simulink model "JenaFox_NCm_visualisation"  (R2018a)
settings: Solver=ode23s  StartTime=0.0  StopTime=20  MaxStep=maxStep  RelTol=1e-3  AbsTol=absTol
values from neighbouring files (symbols this model uses):
  amplifier = 2.28    [init_motor_parameters.m]
  c_coupling_hip = 7/hip_Ra*hip_k/hip_i    (= 1.22844788155)    [init_motor_parameters.m]
  c_coupling_knee = 7/knee_Ra*knee_k/knee_i    (= 0.698088436179)    [init_motor_parameters.m]
  c_hs = 0.1    [Fox_param.m]
  d_coupling_knee = 0.5    [init_motor_parameters.m]
  d_hs = 0.35    [Fox_param.m]
  errorswitch = true    [Fox_param.m]
  g = 9.81    [Fox_param.m]    (also in init_motor_parameters.m)
  hip_i = 1/300.4858    (= 0.00332794428223)    [init_motor_parameters.m]
  hip_Jm = 1/2*hip_m*hip_r^2    (= 1e-07)    [init_motor_parameters.m]
  hip_k = (hip_Um-hip_I0*hip_Ra)*60/(2*pi*hip_n0)    (= 0.00320895298542)    [init_motor_parameters.m]
  hip_Mrg = hip_k*hip_I0g    (= 0.000320895298542)    [init_motor_parameters.m]
  hip_Mrhg = hip_k*hip_Iag    (= 0.000381865405265)    [init_motor_parameters.m]
  hip_na = (hip_Us-(hip_I0*hip_Ra))/hip_k    (= 105.13168591)    [init_motor_parameters.m]
  hip_Ra = hip_Um/hip_Is    (= 5.49450549451)    [init_motor_parameters.m]
  IC_motor_hip_l = deg2rad(IC_phi_hip_l/hip_i)    [init_motor_parameters.m]
  IC_motor_hip_r = deg2rad(IC_phi_hip_r/hip_i)    [init_motor_parameters.m]
  IC_motor_knee_l = deg2rad(IC_phi_knee_l/knee_i)    [init_motor_parameters.m]
  IC_motor_knee_r = deg2rad(IC_phi_knee_r/knee_i)    [init_motor_parameters.m]
  IC_phi_hip_l = 10    [Fox_param.m]
  IC_phi_hip_r = -29    [Fox_param.m]
  IC_v_motor_hip = 0    [init_motor_parameters.m]
  IC_v_motor_knee = 0    [init_motor_parameters.m]
  k_gx = 10*M_RB/0.01    [Fox_param.m]
  k_gy = 150*M_RB/0.01    [Fox_param.m]
  knee_i = 1/185.8428    (= 0.00538089180748)    [init_motor_parameters.m]
  knee_Jm = 1/2*knee_m*knee_r^2    (= 3.2e-08)    [init_motor_parameters.m]
  knee_k = (knee_Um-knee_I0*knee_Ra)*60/(2*pi*knee_n0)    (= 0.000596244182085)    [init_motor_parameters.m]
  knee_Mrg = knee_k*knee_I0g    (= 6.55868600293e-05)    [init_motor_parameters.m]
  knee_Mrhg = knee_k*knee_Iag    (= 9.59953133156e-05)    [init_motor_parameters.m]
  knee_na = (knee_Us-knee_I0*knee_Ra)/knee_k    (= 1360.36733855)    [init_motor_parameters.m]
  knee_Ra = knee_Um/knee_Is    (= 1.11111111111)    [init_motor_parameters.m]
  mu_slide = 4.6    [Fox_param.m]
  mu_stick = 0.8    [Fox_param.m]
  stop5m = true    [Fox_param.m]
  v_gx_max = 0.06    [Fox_param.m]
  v_gy_max = 0.70    (= 0.7)    [Fox_param.m]
  vLimit = 0.01    [Fox_param.m]
undefined symbols (not defined in the file or in its folder): param, smiData, X, Y, Z
libraries: sm_lib x38, nesl_utility x32, simulink x22, simulink_extras x8
(part 2 of 3)

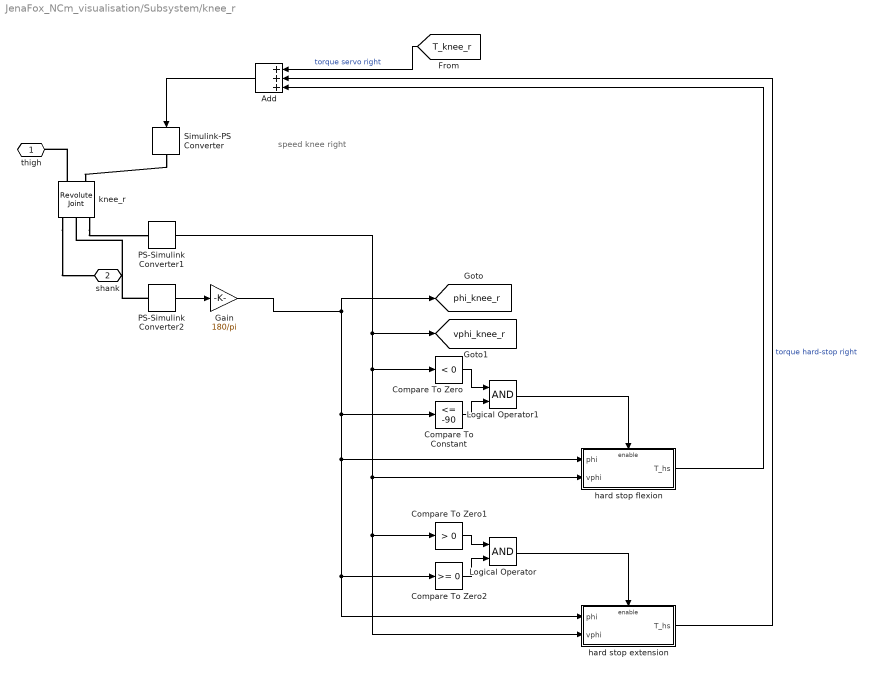
== system JenaFox_NCm_visualisation/Subsystem/knee_r ==
  note: speed knee right
  Add : Sum  Inputs=+++
  Compare To Constant : simulink/Logic and Bit Operations/Compare To Constant  relop=<=  const=-90  OutDataTypeStr=uint8
  Compare To Zero : simulink/Logic and Bit Operations/Compare To Zero  relop=<  OutDataTypeStr=uint8  ZeroCross=off
  Compare To Zero1 : simulink/Logic and Bit Operations/Compare To Zero  relop=>  OutDataTypeStr=uint8  ZeroCross=off
  Compare To Zero2 : simulink/Logic and Bit Operations/Compare To Zero  relop=>=  OutDataTypeStr=uint8
  Gain : Gain  Gain=180/pi
  Logical Operator : Logic  AllPortsSameDT=off  OutDataTypeStr=boolean
  Logical Operator1 : Logic  AllPortsSameDT=off  OutDataTypeStr=boolean
  PS-Simulink Converter1 : nesl_utility/PS-Simulink Converter  PhysicalDomain=network_engine_domain  SubClassName=ps_output  LeftPortType=input  RightPortType=output  PseudoPeriodic=off  Frequencies=[]  Unit=1  AffineConversion=off
  PS-Simulink Converter2 : nesl_utility/PS-Simulink Converter  PhysicalDomain=network_engine_domain  SubClassName=ps_output  LeftPortType=input  RightPortType=output  PseudoPeriodic=off  Frequencies=[]  Unit=1  AffineConversion=off
  Simulink-PS Converter : nesl_utility/Simulink-PS Converter  PhysicalDomain=network_engine_domain  SubClassName=ps_input  LeftPortType=input  RightPortType=output  PseudoPeriodic=off  Frequencies=[]  NoiseDistribution=none  NoiseParameters=[]  Unit=1  AffineConversion=off  FilteringAndDerivatives=provide  SimscapeFilterOrder=1  InputFilterTimeConstant=0.001  UdotUserProvided=0
  hard stop extension : Subsystem  TreatAsAtomicUnit=on
  hard stop flexion : Subsystem  TreatAsAtomicUnit=on
  knee_r : sm_lib/Joints/Revolute Joint  SenseConstraintForce=off  SenseConstraintForceX=off  SenseConstraintForceY=off  SenseConstraintForceZ=off  SenseConstraintTorque=off  SenseConstraintTorqueX=off  SenseConstraintTorqueY=off  SenseConstraintTorqueZ=off  SenseTotalForce=off  SenseTotalForceX=off  SenseTotalForceY=off  SenseTotalForceZ=off  SenseTotalTorque=off  SenseTotalTorqueX=off  SenseTotalTorqueY=off  SenseTotalTorqueZ=off  CompositeWrenchDir=FollowerOnBase  CompositeWrenchFrame=BaseFrame  EquilibriumPosition=0  EquilibriumPositionUnits=rad  SpringStiffness=0  SpringStiffnessUnits=N*m/rad  DampingCoefficient=d_joint  DampingCoefficientUnits=N*m/(rad/s)  TorqueActuationMode=InputTorque  MotionActuationMode=ComputedMotion  SensePosition=on  SenseVelocity=on  SenseAcceleration=off  SenseTorqueForce=off  PositionTargetSpecify=on  PositionTargetPriority=High  PositionTargetValue=IC_phi_knee_r  PositionTargetValueUnits=deg  VelocityTargetSpecify=off  VelocityTargetPriority=High  VelocityTargetValue=0  VelocityTargetValueUnits=deg/s
  thigh : PMIOPort  Side=Left
  shank : PMIOPort  Port=2  Side=Right
  tag scope: phi_knee_r=global, vphi_knee_r=global
  wires:
  Compare To Constant/1 -> Logical Operator1/2
  PS-Simulink Converter2/1 -> Gain/1
  hard stop extension/1(T_hs) -> Add/2  "torque hard-stop right"
  Compare To Zero1/1 -> Logical Operator/1
  Logical Operator1/1 -> hard stop flexion/Enable
  Logical Operator/1 -> hard stop extension/Enable
  Add/1 -> Simulink-PS Converter/1
  Compare To Zero/1 -> Logical Operator1/1
  PS-Simulink Converter1/1 -> [vphi_knee_r], Compare To Zero/1, hard stop flexion/2(vphi), Compare To Zero1/1, hard stop extension/2(vphi)
  hard stop flexion/1(T_hs) -> Add/3
  Compare To Zero2/1 -> Logical Operator/2
  [T_knee_r] -> Add/1  "torque servo right"
  Gain/1 -> [phi_knee_r], Compare To Constant/1, hard stop flexion/1(phi), Compare To Zero2/1, hard stop extension/1(phi)
  connections:
  Simulink-PS Converter/RConn1 -- knee_r/LConn2
  knee_r/RConn1 -- shank/RConn1
  PS-Simulink Converter2/LConn1 -- knee_r/RConn2
  knee_r/RConn3 -- PS-Simulink Converter1/LConn1
  knee_r/LConn1 -- thigh/RConn1

== system JenaFox_NCm_visualisation/Subsystem/shank_bottom_l ==
  Rigid Transform : sm_lib/Frames and Transforms/Rigid Transform  TranslationMethod=None  TranslationStandardOffset=0  TranslationLengthUnit=m  TranslationStandardAxis=+Z  TranslationCartesianOffset=[0 0 0]  TranslationROffset=0  TranslationROffsetUnits=m  TranslationZOffset=0  TranslationZOffsetUnits=m  TranslationThetaOffset=0  TranslationThetaOffsetUnits=deg  RotationMethod=AlignedAxes  RotationAngleUnits=deg  RotationStandardAxis=+Z  RotationAngle=0.0  RotationArbitraryAxis=[0 0 1]  FollAlignAxisA=+X  BaseAlignAxisA=-X  FollAlignAxisB=+Z  BaseAlignAxisB=+Y  RotationSequenceAxes=FollowerAxes  RotationSequence=XYX  RotationSequenceAngles=[0 0 0]  RotationSequenceAnglesUnits=deg  RotationMatrix=[1 0 0; 0 1 0; 0 0 1]
  Solid : sm_lib/Body Elements/Solid  InertiaType=Custom  Mass=smiData.Solid(4).mass  MassUnits=kg  CenterOfMass=smiData.Solid(4).CoM  CenterOfMassUnits=mm  MomentsOfInertia=smiData.Solid(4).MoI  MomentsOfInertiaUnits=kg*mm^2  ProductsOfInertia=smiData.Solid(4).PoI  ProductsOfInertiaUnits=kg*mm^2  DensityBased=on  Density=1000  DensityUnits=kg/m^3  DoExposeReferenceFrame=on  SerializedFrames=<Frames><Frame><Id>Frame1</Id><Value><Name>ground_contact</Name><Origin><Source>GeometricFeature</Source><FeatureName>circular curve 105</FeatureName></Origin><PrimaryAxis><DefinedDirection>+Y</DefinedDirection><Source>ReferenceFrame</Source><SourceDirection>-Y</SourceDirection><FeatureName></FeatureName></PrimaryAxis><SecondaryAxis><DefinedDirection>+X</DefinedDirection><Source>ReferenceFrame</Source><SourceDirection>+X</SourceDirection><FeatureName></FeatureName></SecondaryAxis></Value></Frame><Frame><Id>Frame2</Id><Value><Name>spring_bottom</Name><Origin><Source>GeometricFeature</Source><FeatureName>circular curve 81</FeatureName></Origin><PrimaryAxis><DefinedDirection>+Y</DefinedDirection><Source>ReferenceFrame</Source><SourceDirection>-Y</SourceDirection><FeatureName></FeatureName></PrimaryAxis><SecondaryAxis><DefinedDirection>+X</DefinedDirection><Source>ReferenceFrame</Source><SourceDirection>+X</SourceDirection><FeatureName></FeatureName></SecondaryAxis></Value></Frame></Frames>  GraphicType=FromGeometry  MarkerShape=Sphere  MarkerSize=10  GraphicVisPropType=SimpleVisualProperties  GraphicDiffuseColor=smiData.Solid(4).color  GraphicSpecularColor=[0.5 0.5 0.5 1.0]  GraphicAmbientColor=[0.15 0.15 0.15 1.0]  GraphicEmissiveColor=[0.0 0.0 0.0 1.0]  GraphicShininess=75  GraphicOpacity=smiData.Solid(4).opacity  GeometryShape=FromFile  RectangleSize=[1 1]  RectangleSizeUnits=m  BrickDimensions=[1 1 1]  BrickDimensionUnits=m  CylinderRadius=1  CylinderRadiusUnits=m  CylinderLength=1  CylinderLengthUnits=m  SphereRadius=1  SphereRadiusUnits=m  EllipsoidRadii=[1 1 1]  EllipsoidRadiiUnits=m  ExtrusionCrossSection=[1 1; -1 1; -1 -1; 1 -1]  ExtrusionCrossSectionUnits=m  ExtrusionLength=1  ExtrusionLengthUnits=m  PolygonNumSides=3  PolygonOuterRadius=1  PolygonOuterRadiusUnits=m  ExtGeomFileType=STEP  ExtGeomFileName=shank_bottom_ipt_92530788.STEP  ExtGeomFileUnits=m  RevolutionCrossSection=[1 1; 1 -1; 2 -1; 2 1]  RevolutionCrossSectionUnits=m  RevolutionExtent=Full  RevolutionAngle=180  RevolutionAngleUnits=deg
  linear elastic joint : PMIOPort  Side=Left
  toe : PMIOPort  Port=2  Side=Right
  spring_bottom : PMIOPort  Port=3  Side=Left
  connections:
  toe/RConn1 -- Solid/LConn1
  linear elastic joint/RConn1 -- Rigid Transform/RConn1 -- spring_bottom/RConn1
  Rigid Transform/LConn1 -- Solid/LConn2

== system JenaFox_NCm_visualisation/Subsystem/shank_bottom_r ==
  Rigid Transform : sm_lib/Frames and Transforms/Rigid Transform  TranslationMethod=None  TranslationStandardOffset=0  TranslationLengthUnit=m  TranslationStandardAxis=+Z  TranslationCartesianOffset=[0 0 0]  TranslationROffset=0  TranslationROffsetUnits=m  TranslationZOffset=0  TranslationZOffsetUnits=m  TranslationThetaOffset=0  TranslationThetaOffsetUnits=deg  RotationMethod=AlignedAxes  RotationAngleUnits=deg  RotationStandardAxis=+Z  RotationAngle=0.0  RotationArbitraryAxis=[0 0 1]  FollAlignAxisA=+X  BaseAlignAxisA=+X  FollAlignAxisB=+Z  BaseAlignAxisB=+Y  RotationSequenceAxes=FollowerAxes  RotationSequence=XYX  RotationSequenceAngles=[0 0 0]  RotationSequenceAnglesUnits=deg  RotationMatrix=[1 0 0; 0 1 0; 0 0 1]
  Solid : sm_lib/Body Elements/Solid  InertiaType=Custom  Mass=smiData.Solid(4).mass  MassUnits=kg  CenterOfMass=smiData.Solid(4).CoM  CenterOfMassUnits=mm  MomentsOfInertia=smiData.Solid(4).MoI  MomentsOfInertiaUnits=kg*mm^2  ProductsOfInertia=smiData.Solid(4).PoI  ProductsOfInertiaUnits=kg*mm^2  DensityBased=on  Density=1000  DensityUnits=kg/m^3  DoExposeReferenceFrame=off  SerializedFrames=<Frames><Frame><Id>Frame1</Id><Value><Name>ground_contact</Name><Origin><Source>GeometricFeature</Source><FeatureName>circular curve 105</FeatureName></Origin><PrimaryAxis><DefinedDirection>+Y</DefinedDirection><Source>ReferenceFrame</Source><SourceDirection>-Y</SourceDirection><FeatureName></FeatureName></PrimaryAxis><SecondaryAxis><DefinedDirection>+X</DefinedDirection><Source>ReferenceFrame</Source><SourceDirection>+X</SourceDirection><FeatureName></FeatureName></SecondaryAxis></Value></Frame><Frame><Id>Frame2</Id><Value><Name>spring_bottom</Name><Origin><Source>GeometricFeature</Source><FeatureName>circular curve 81</FeatureName></Origin><PrimaryAxis><DefinedDirection>+Y</DefinedDirection><Source>ReferenceFrame</Source><SourceDirection>-Y</SourceDirection><FeatureName></FeatureName></PrimaryAxis><SecondaryAxis><DefinedDirection>+X</DefinedDirection><Source>ReferenceFrame</Source><SourceDirection>+X</SourceDirection><FeatureName></FeatureName></SecondaryAxis></Value></Frame></Frames>  GraphicType=FromGeometry  MarkerShape=Sphere  MarkerSize=10  GraphicVisPropType=SimpleVisualProperties  GraphicDiffuseColor=smiData.Solid(4).color  GraphicSpecularColor=[0.5 0.5 0.5 1.0]  GraphicAmbientColor=[0.15 0.15 0.15 1.0]  GraphicEmissiveColor=[0.0 0.0 0.0 1.0]  GraphicShininess=75  GraphicOpacity=smiData.Solid(4).opacity  GeometryShape=FromFile  RectangleSize=[1 1]  RectangleSizeUnits=m  BrickDimensions=[1 1 1]  BrickDimensionUnits=m  CylinderRadius=1  CylinderRadiusUnits=m  CylinderLength=1  CylinderLengthUnits=m  SphereRadius=1  SphereRadiusUnits=m  EllipsoidRadii=[1 1 1]  EllipsoidRadiiUnits=m  ExtrusionCrossSection=[1 1; -1 1; -1 -1; 1 -1]  ExtrusionCrossSectionUnits=m  ExtrusionLength=1  ExtrusionLengthUnits=m  PolygonNumSides=3  PolygonOuterRadius=1  PolygonOuterRadiusUnits=m  ExtGeomFileType=STEP  ExtGeomFileName=shank_bottom_ipt_92530788.STEP  ExtGeomFileUnits=m  RevolutionCrossSection=[1 1; 1 -1; 2 -1; 2 1]  RevolutionCrossSectionUnits=m  RevolutionExtent=Full  RevolutionAngle=180  RevolutionAngleUnits=deg
  linear elastic joint : PMIOPort  Side=Left
  toe : PMIOPort  Port=2  Side=Right
  spring_bottom : PMIOPort  Port=3  Side=Left
  connections:
  toe/RConn1 -- Solid/LConn1
  linear elastic joint/RConn1 -- Rigid Transform/RConn1 -- spring_bottom/RConn1
  Rigid Transform/LConn1 -- Solid/RConn1

== system JenaFox_NCm_visualisation/Subsystem/shank_top_l ==
  Rigid Transform : sm_lib/Frames and Transforms/Rigid Transform  TranslationMethod=StandardAxis  TranslationStandardOffset=0.11  TranslationLengthUnit=m  TranslationStandardAxis=+Z  TranslationCartesianOffset=[0 0 0]  TranslationROffset=0  TranslationROffsetUnits=m  TranslationZOffset=0  TranslationZOffsetUnits=m  TranslationThetaOffset=0  TranslationThetaOffsetUnits=deg  RotationMethod=AlignedAxes  RotationAngleUnits=deg  RotationStandardAxis=+Z  RotationAngle=0.0  RotationArbitraryAxis=[0 0 1]  FollAlignAxisA=+X  BaseAlignAxisA=+X  FollAlignAxisB=+Y  BaseAlignAxisB=+Z  RotationSequenceAxes=FollowerAxes  RotationSequence=XYX  RotationSequenceAngles=[0 0 0]  RotationSequenceAnglesUnits=deg  RotationMatrix=[1 0 0; 0 1 0; 0 0 1]
  Solid : sm_lib/Body Elements/Solid  InertiaType=Custom  Mass=smiData.Solid(3).mass  MassUnits=kg  CenterOfMass=smiData.Solid(3).CoM  CenterOfMassUnits=mm  MomentsOfInertia=smiData.Solid(3).MoI  MomentsOfInertiaUnits=kg*mm^2  ProductsOfInertia=smiData.Solid(3).PoI  ProductsOfInertiaUnits=kg*mm^2  DensityBased=on  Density=1000  DensityUnits=kg/m^3  DoExposeReferenceFrame=off  SerializedFrames=<Frames><Frame><Id>Frame1</Id><Value><Name>spring_top</Name><Origin><Source>GeometricFeature</Source><FeatureName>circular curve 166</FeatureName></Origin><PrimaryAxis><DefinedDirection>+Y</DefinedDirection><Source>ReferenceFrame</Source><SourceDirection>-Y</SourceDirection><FeatureName></FeatureName></PrimaryAxis><SecondaryAxis><DefinedDirection>+X</DefinedDirection><Source>GeometricFeature</Source><SourceDirection>+X</SourceDirection><FeatureName>segment 110</FeatureName></SecondaryAxis></Value></Frame><Frame><Id>Frame2</Id><Value><Name>knee</Name><Origin><Source>GeometricFeature</Source><FeatureName>circular curve 135</FeatureName></Origin><PrimaryAxis><DefinedDirection>-X</DefinedDirection><Source>GeometricFeature</Source><SourceDirection>+Z</SourceDirection><FeatureName>segment 80</FeatureName></PrimaryAxis><SecondaryAxis><DefinedDirection>+Y</DefinedDirection><Source>GeometricFeature</Source><SourceDirection>+X</SourceDirection><FeatureName>segment 115</FeatureName></SecondaryAxis></Value></Frame></Frames>  GraphicType=FromGeometry  MarkerShape=Sphere  MarkerSize=10  GraphicVisPropType=SimpleVisualProperties  GraphicDiffuseColor=smiData.Solid(3).color  GraphicSpecularColor=[0.5 0.5 0.5 1.0]  GraphicAmbientColor=[0.15 0.15 0.15 1.0]  GraphicEmissiveColor=[0.0 0.0 0.0 1.0]  GraphicShininess=75  GraphicOpacity=smiData.Solid(3).opacity  GeometryShape=FromFile  RectangleSize=[1 1]  RectangleSizeUnits=m  BrickDimensions=[1 1 1]  BrickDimensionUnits=m  CylinderRadius=1  CylinderRadiusUnits=m  CylinderLength=1  CylinderLengthUnits=m  SphereRadius=1  SphereRadiusUnits=m  EllipsoidRadii=[1 1 1]  EllipsoidRadiiUnits=m  ExtrusionCrossSection=[1 1; -1 1; -1 -1; 1 -1]  ExtrusionCrossSectionUnits=m  ExtrusionLength=1  ExtrusionLengthUnits=m  PolygonNumSides=3  PolygonOuterRadius=1  PolygonOuterRadiusUnits=m  ExtGeomFileType=STEP  ExtGeomFileName=shank_top_ipt_5be12039.STEP  ExtGeomFileUnits=m  RevolutionCrossSection=[1 1; 1 -1; 2 -1; 2 1]  RevolutionCrossSectionUnits=m  RevolutionExtent=Full  RevolutionAngle=180  RevolutionAngleUnits=deg
  knee : PMIOPort  Side=Left
  linear joint : PMIOPort  Port=2  Side=Right
  spring_top : PMIOPort  Port=3  Side=Right
  connections:
  knee/RConn1 -- Solid/RConn1
  Rigid Transform/RConn1 -- spring_top/RConn1 -- Solid/LConn1
  linear joint/RConn1 -- Rigid Transform/LConn1

== system JenaFox_NCm_visualisation/Subsystem/shank_top_r ==
  Rigid Transform : sm_lib/Frames and Transforms/Rigid Transform  TranslationMethod=StandardAxis  TranslationStandardOffset=0.11  TranslationLengthUnit=m  TranslationStandardAxis=+Z  TranslationCartesianOffset=[0 0 0]  TranslationROffset=0  TranslationROffsetUnits=m  TranslationZOffset=0  TranslationZOffsetUnits=m  TranslationThetaOffset=0  TranslationThetaOffsetUnits=deg  RotationMethod=AlignedAxes  RotationAngleUnits=deg  RotationStandardAxis=+Z  RotationAngle=0.0  RotationArbitraryAxis=[0 0 1]  FollAlignAxisA=+X  BaseAlignAxisA=+X  FollAlignAxisB=+Y  BaseAlignAxisB=+Z  RotationSequenceAxes=FollowerAxes  RotationSequence=XYX  RotationSequenceAngles=[0 0 0]  RotationSequenceAnglesUnits=deg  RotationMatrix=[1 0 0; 0 1 0; 0 0 1]
  Solid : sm_lib/Body Elements/Solid  InertiaType=Custom  Mass=smiData.Solid(3).mass  MassUnits=kg  CenterOfMass=smiData.Solid(3).CoM  CenterOfMassUnits=mm  MomentsOfInertia=smiData.Solid(3).MoI  MomentsOfInertiaUnits=kg*mm^2  ProductsOfInertia=smiData.Solid(3).PoI  ProductsOfInertiaUnits=kg*mm^2  DensityBased=on  Density=1000  DensityUnits=kg/m^3  DoExposeReferenceFrame=off  SerializedFrames=<Frames><Frame><Id>Frame1</Id><Value><Name>spring_top</Name><Origin><Source>GeometricFeature</Source><FeatureName>circular curve 166</FeatureName></Origin><PrimaryAxis><DefinedDirection>+Y</DefinedDirection><Source>ReferenceFrame</Source><SourceDirection>-Y</SourceDirection><FeatureName></FeatureName></PrimaryAxis><SecondaryAxis><DefinedDirection>+X</DefinedDirection><Source>GeometricFeature</Source><SourceDirection>+X</SourceDirection><FeatureName>segment 110</FeatureName></SecondaryAxis></Value></Frame><Frame><Id>Frame2</Id><Value><Name>shank_knee_right</Name><Origin><Source>GeometricFeature</Source><FeatureName>circular curve 135</FeatureName></Origin><PrimaryAxis><DefinedDirection>+X</DefinedDirection><Source>GeometricFeature</Source><SourceDirection>+Z</SourceDirection><FeatureName>segment 110</FeatureName></PrimaryAxis><SecondaryAxis><DefinedDirection>+Y</DefinedDirection><Source>GeometricFeature</Source><SourceDirection>+X</SourceDirection><FeatureName>segment 138</FeatureName></SecondaryAxis></Value></Frame></Frames>  GraphicType=FromGeometry  MarkerShape=Sphere  MarkerSize=10  GraphicVisPropType=SimpleVisualProperties  GraphicDiffuseColor=smiData.Solid(3).color  GraphicSpecularColor=[0.5 0.5 0.5 1.0]  GraphicAmbientColor=[0.15 0.15 0.15 1.0]  GraphicEmissiveColor=[0.0 0.0 0.0 1.0]  GraphicShininess=75  GraphicOpacity=smiData.Solid(3).opacity  GeometryShape=FromFile  RectangleSize=[1 1]  RectangleSizeUnits=m  BrickDimensions=[1 1 1]  BrickDimensionUnits=m  CylinderRadius=1  CylinderRadiusUnits=m  CylinderLength=1  CylinderLengthUnits=m  SphereRadius=1  SphereRadiusUnits=m  EllipsoidRadii=[1 1 1]  EllipsoidRadiiUnits=m  ExtrusionCrossSection=[1 1; -1 1; -1 -1; 1 -1]  ExtrusionCrossSectionUnits=m  ExtrusionLength=1  ExtrusionLengthUnits=m  PolygonNumSides=3  PolygonOuterRadius=1  PolygonOuterRadiusUnits=m  ExtGeomFileType=STEP  ExtGeomFileName=shank_top_ipt_5be12039.STEP  ExtGeomFileUnits=m  RevolutionCrossSection=[1 1; 1 -1; 2 -1; 2 1]  RevolutionCrossSectionUnits=m  RevolutionExtent=Full  RevolutionAngle=180  RevolutionAngleUnits=deg
  knee : PMIOPort  Side=Left
  linear joint : PMIOPort  Port=2  Side=Right
  spring_top : PMIOPort  Port=3  Side=Right
  connections:
  knee/RConn1 -- Solid/RConn1
  Rigid Transform/RConn1 -- spring_top/RConn1 -- Solid/LConn1
  linear joint/RConn1 -- Rigid Transform/LConn1

== system JenaFox_NCm_visualisation/Subsystem/simulation terminator ==
  Clock : Clock
  PS-Simulink Converter : nesl_utility/PS-Simulink Converter  PhysicalDomain=network_engine_domain  SubClassName=ps_output  LeftPortType=input  RightPortType=output  PseudoPeriodic=off  Frequencies=[]  Unit=1  AffineConversion=off
  PS-Simulink Converter1 : nesl_utility/PS-Simulink Converter  PhysicalDomain=network_engine_domain  SubClassName=ps_output  LeftPortType=input  RightPortType=output  PseudoPeriodic=off  Frequencies=[]  Unit=1  AffineConversion=off
  PS-Simulink Converter2 : nesl_utility/PS-Simulink Converter  PhysicalDomain=network_engine_domain  SubClassName=ps_output  LeftPortType=input  RightPortType=output  PseudoPeriodic=off  Frequencies=[]  Unit=1  AffineConversion=off
  Subsystem : Subsystem
  error handling : Subsystem
  time of termination : Subsystem
  x : PMIOPort  Side=Left
  y : PMIOPort  Port=2  Side=Left
  dx : PMIOPort  Port=3  Side=Left
  wires:
  error handling/1(error) -> Subsystem/1(error), time of termination/1(error)
  PS-Simulink Converter/1 -> Subsystem/2(x), time of termination/3(x)  "x"
  PS-Simulink Converter1/1 -> error handling/3(dx)
  Clock/1 -> time of termination/2(t), error handling/1(t)
  PS-Simulink Converter2/1 -> error handling/2(y)
  connections:
  PS-Simulink Converter/LConn1 -- x/RConn1
  PS-Simulink Converter1/LConn1 -- dx/RConn1
  PS-Simulink Converter2/LConn1 -- y/RConn1

== system JenaFox_NCm_visualisation/Subsystem/thigh_l ==
  Solid : sm_lib/Body Elements/Solid  InertiaType=Custom  Mass=smiData.Solid(2).mass  MassUnits=kg  CenterOfMass=smiData.Solid(2).CoM  CenterOfMassUnits=mm  MomentsOfInertia=smiData.Solid(2).MoI  MomentsOfInertiaUnits=kg*mm^2  ProductsOfInertia=smiData.Solid(2).PoI  ProductsOfInertiaUnits=kg*mm^2  DensityBased=on  Density=1000  DensityUnits=kg/m^3  DoExposeReferenceFrame=off  SerializedFrames=<Frames><Frame><Id>Frame1</Id><Value><Name>thigh_left_knee</Name><Origin><Source>GeometricFeature</Source><FeatureName>planar surface 172</FeatureName></Origin><PrimaryAxis><DefinedDirection>+Z</DefinedDirection><Source>ReferenceFrame</Source><SourceDirection>-Y</SourceDirection><FeatureName></FeatureName></PrimaryAxis><SecondaryAxis><DefinedDirection>+X</DefinedDirection><Source>ReferenceFrame</Source><SourceDirection>+X</SourceDirection><FeatureName></FeatureName></SecondaryAxis></Value></Frame><Frame><Id>Frame2</Id><Value><Name>thigh_left_hip</Name><Origin><Source>GeometricFeature</Source><FeatureName>circular curve 156</FeatureName></Origin><PrimaryAxis><DefinedDirection>+Z</DefinedDirection><Source>ReferenceFrame</Source><SourceDirection>-Y</SourceDirection><FeatureName></FeatureName></PrimaryAxis><SecondaryAxis><DefinedDirection>+X</DefinedDirection><Source>ReferenceFrame</Source><SourceDirection>+X</SourceDirection><FeatureName></FeatureName></SecondaryAxis></Value></Frame></Frames>  GraphicType=FromGeometry  MarkerShape=Sphere  MarkerSize=10  GraphicVisPropType=SimpleVisualProperties  GraphicDiffuseColor=smiData.Solid(2).color  GraphicSpecularColor=[0.5 0.5 0.5 1.0]  GraphicAmbientColor=[0.15 0.15 0.15 1.0]  GraphicEmissiveColor=[0.0 0.0 0.0 1.0]  GraphicShininess=75  GraphicOpacity=smiData.Solid(2).opacity  GeometryShape=FromFile  RectangleSize=[1 1]  RectangleSizeUnits=m  BrickDimensions=[1 1 1]  BrickDimensionUnits=m  CylinderRadius=1  CylinderRadiusUnits=m  CylinderLength=1  CylinderLengthUnits=m  SphereRadius=1  SphereRadiusUnits=m  EllipsoidRadii=[1 1 1]  EllipsoidRadiiUnits=m  ExtrusionCrossSection=[1 1; -1 1; -1 -1; 1 -1]  ExtrusionCrossSectionUnits=m  ExtrusionLength=1  ExtrusionLengthUnits=m  PolygonNumSides=3  PolygonOuterRadius=1  PolygonOuterRadiusUnits=m  ExtGeomFileType=STEP  ExtGeomFileName=thigh_left_ipt_d01cdd9b.STEP  ExtGeomFileUnits=m  RevolutionCrossSection=[1 1; 1 -1; 2 -1; 2 1]  RevolutionCrossSectionUnits=m  RevolutionExtent=Full  RevolutionAngle=180  RevolutionAngleUnits=deg
  hip : PMIOPort  Side=Left
  knee : PMIOPort  Port=2  Side=Right
  connections:
  hip/RConn1 -- Solid/RConn1
  knee/RConn1 -- Solid/LConn1

== system JenaFox_NCm_visualisation/Subsystem/thigh_r ==
  Solid : sm_lib/Body Elements/Solid  InertiaType=Custom  Mass=smiData.Solid(2).mass  MassUnits=kg  CenterOfMass=smiData.Solid(2).CoM  CenterOfMassUnits=mm  MomentsOfInertia=smiData.Solid(2).MoI  MomentsOfInertiaUnits=kg*mm^2  ProductsOfInertia=smiData.Solid(2).PoI  ProductsOfInertiaUnits=kg*mm^2  DensityBased=on  Density=1000  DensityUnits=kg/m^3  DoExposeReferenceFrame=off  SerializedFrames=<Frames><Frame><Id>Frame1</Id><Value><Name>thigh_right_knee</Name><Origin><Source>GeometricFeature</Source><FeatureName>circular curve 616</FeatureName></Origin><PrimaryAxis><DefinedDirection>+Z</DefinedDirection><Source>ReferenceFrame</Source><SourceDirection>+Y</SourceDirection><FeatureName></FeatureName></PrimaryAxis><SecondaryAxis><DefinedDirection>+X</DefinedDirection><Source>ReferenceFrame</Source><SourceDirection>-X</SourceDirection><FeatureName></FeatureName></SecondaryAxis></Value></Frame><Frame><Id>Frame2</Id><Value><Name>thigh_right_hip</Name><Origin><Source>GeometricFeature</Source><FeatureName>circular curve 280</FeatureName></Origin><PrimaryAxis><DefinedDirection>+Z</DefinedDirection><Source>ReferenceFrame</Source><SourceDirection>+Y</SourceDirection><FeatureName></FeatureName></PrimaryAxis><SecondaryAxis><DefinedDirection>+X</DefinedDirection><Source>ReferenceFrame</Source><SourceDirection>-X</SourceDirection><FeatureName></FeatureName></SecondaryAxis></Value></Frame></Frames>  GraphicType=FromGeometry  MarkerShape=Sphere  MarkerSize=10  GraphicVisPropType=SimpleVisualProperties  GraphicDiffuseColor=smiData.Solid(2).color  GraphicSpecularColor=[0.5 0.5 0.5 1.0]  GraphicAmbientColor=[0.15 0.15 0.15 1.0]  GraphicEmissiveColor=[0.0 0.0 0.0 1.0]  GraphicShininess=75  GraphicOpacity=smiData.Solid(2).opacity  GeometryShape=FromFile  RectangleSize=[1 1]  RectangleSizeUnits=m  BrickDimensions=[1 1 1]  BrickDimensionUnits=m  CylinderRadius=1  CylinderRadiusUnits=m  CylinderLength=1  CylinderLengthUnits=m  SphereRadius=1  SphereRadiusUnits=m  EllipsoidRadii=[1 1 1]  EllipsoidRadiiUnits=m  ExtrusionCrossSection=[1 1; -1 1; -1 -1; 1 -1]  ExtrusionCrossSectionUnits=m  ExtrusionLength=1  ExtrusionLengthUnits=m  PolygonNumSides=3  PolygonOuterRadius=1  PolygonOuterRadiusUnits=m  ExtGeomFileType=STEP  ExtGeomFileName=thigh_left_ipt_d01cdd9b.STEP  ExtGeomFileUnits=m  RevolutionCrossSection=[1 1; 1 -1; 2 -1; 2 1]  RevolutionCrossSectionUnits=m  RevolutionExtent=Full  RevolutionAngle=180  RevolutionAngleUnits=deg
  hip : PMIOPort  Side=Left
  knee : PMIOPort  Port=2  Side=Right
  connections:
  knee/RConn1 -- Solid/LConn1
  Solid/RConn1 -- hip/RConn1

== system JenaFox_NCm_visualisation/Subsystem/trunk ==
  Solid : sm_lib/Body Elements/Solid  InertiaType=Custom  Mass=smiData.Solid(1).mass  MassUnits=kg  CenterOfMass=smiData.Solid(1).CoM  CenterOfMassUnits=mm  MomentsOfInertia=smiData.Solid(1).MoI  MomentsOfInertiaUnits=kg*mm^2  ProductsOfInertia=smiData.Solid(1).PoI  ProductsOfInertiaUnits=kg*mm^2  DensityBased=on  Density=1000  DensityUnits=kg/m^3  DoExposeReferenceFrame=off  SerializedFrames=<Frames><Frame><Id>Frame1</Id><Value><Name>hip_right</Name><Origin><Source>GeometricFeature</Source><FeatureName>circular curve 591</FeatureName></Origin><PrimaryAxis><DefinedDirection>+Z</DefinedDirection><Source>ReferenceFrame</Source><SourceDirection>+X</SourceDirection><FeatureName></FeatureName></PrimaryAxis><SecondaryAxis><DefinedDirection>+X</DefinedDirection><Source>ReferenceFrame</Source><SourceDirection>-Z</SourceDirection><FeatureName></FeatureName></SecondaryAxis></Value></Frame><Frame><Id>Frame2</Id><Value><Name>hip_left</Name><Origin><Source>GeometricFeature</Source><FeatureName>circular curve 612</FeatureName></Origin><PrimaryAxis><DefinedDirection>+Z</DefinedDirection><Source>ReferenceFrame</Source><SourceDirection>+X</SourceDirection><FeatureName></FeatureName></PrimaryAxis><SecondaryAxis><DefinedDirection>+X</DefinedDirection><Source>ReferenceFrame</Source><SourceDirection>-Z</SourceDirection><FeatureName></FeatureName></SecondaryAxis></Value></Frame><Frame><Id>Frame3</Id><Value><Name>boom_connector</Name><Origin><Source>GeometricFeature</Source><FeatureName>circular curve 1475</FeatureName></Origin><PrimaryAxis><DefinedDirection>+X</DefinedDirection><Source>ReferenceFrame</Source><SourceDirection>-Z</SourceDirection><FeatureName></FeatureName></PrimaryAxis><SecondaryAxis><DefinedDirection>+Y</DefinedDirection><Source>ReferenceFrame</Source><SourceDirection>+Y</SourceDirection><FeatureName></FeatureName></SecondaryAxis></Value></Frame></Frames>  GraphicType=FromGeometry  MarkerShape=Sphere  MarkerSize=10  GraphicVisPropType=SimpleVisualProperties  GraphicDiffuseColor=smiData.Solid(1).color  GraphicSpecularColor=[0.5 0.5 0.5 1.0]  GraphicAmbientColor=[0.15 0.15 0.15 1.0]  GraphicEmissiveColor=[0.0 0.0 0.0 1.0]  GraphicShininess=75  GraphicOpacity=smiData.Solid(1).opacity  GeometryShape=FromFile  RectangleSize=[1 1]  RectangleSizeUnits=m  BrickDimensions=[1 1 1]  BrickDimensionUnits=m  CylinderRadius=1  CylinderRadiusUnits=m  CylinderLength=1  CylinderLengthUnits=m  SphereRadius=1  SphereRadiusUnits=m  EllipsoidRadii=[1 1 1]  EllipsoidRadiiUnits=m  ExtrusionCrossSection=[1 1; -1 1; -1 -1; 1 -1]  ExtrusionCrossSectionUnits=m  ExtrusionLength=1  ExtrusionLengthUnits=m  PolygonNumSides=3  PolygonOuterRadius=1  PolygonOuterRadiusUnits=m  ExtGeomFileType=STEP  ExtGeomFileName=trunk_ipt_7785b5f2.STEP  ExtGeomFileUnits=m  RevolutionCrossSection=[1 1; 1 -1; 2 -1; 2 1]  RevolutionCrossSectionUnits=m  RevolutionExtent=Full  RevolutionAngle=180  RevolutionAngleUnits=deg
  hip left : PMIOPort  Side=Right
  hip right : PMIOPort  Port=2  Side=Right
  boom : PMIOPort  Port=3  Side=Left
  connections:
  Solid/RConn1 -- hip left/RConn1
  hip right/RConn1 -- Solid/LConn1
  boom/RConn1 -- Solid/LConn2

== system JenaFox_NCm_visualisation/motor model/hip_motor_left ==
  note: IC_phi_motor
  note: IC_v_motor
  note: due to neglectible inductivity the
      | PT1 - transfer function is reduced to an
      | proportional transfer function
      | (Modellbildung und Simulation dynamischer Systeme, S.122)
  U : Inport
  phi_motor : Inport  Port=2
  Add1 : Sum  Inputs=+--
  M_func_hip1 : Lookup  InputValues=[-10^10 -hip_na -0.001 0 0.001 hip_na 10^10]  Table=[-hip_Mrg -hip_Mrg -hip_Mrhg 0 hip_Mrhg hip_Mrg hip_Mrg]
  Radians to Degrees : simulink_extras/Transformations/Radians to Degrees
  Sum1 : Sum  Inputs=|+-
  elastic coupling : Sum  Inputs=+-
  elasticity : Gain  Gain=c_coupling_hip
  gearhead : Gain  Gain=hip_i
  gearhead1 : Gain  Gain=hip_i
  motor constant 1 : Gain  Gain=hip_k
  motor constant1 : Gain  Gain=hip_k
  motor interia : Gain  Gain=1/hip_Jm
  position : Integrator  InitialCondition=IC_motor_hip_l  ContinuousStateAttributes='position_hip'
  rotor resistor1 : Gain  Gain=1/hip_Ra
  speed : Integrator  InitialCondition=IC_v_motor_hip  ContinuousStateAttributes='speed_hip'
  motor_torque : Outport
  current : Outport  Port=2
  wires:
  elasticity/1 -> motor_torque/1, gearhead1/1  "coupling torque"
  gearhead1/1 -> Add1/3
  phi_motor/1 -> elastic coupling/2
  U/1 -> Sum1/1
  Radians to Degrees/1 -> gearhead/1  "position in °"
  gearhead/1 -> elastic coupling/1
  elastic coupling/1 -> elasticity/1
  position/1 -> Radians to Degrees/1  "position"
  motor constant 1/1 -> Sum1/2  "inductive voltage"
  speed/1 -> motor constant 1/1, M_func_hip1/1, position/1  "motor speed"
  Sum1/1 -> rotor resistor1/1
  motor interia/1 -> speed/1  "acceleration"
  Add1/1 -> motor interia/1
  M_func_hip1/1 -> Add1/2  "friction torque"
  motor constant1/1 -> Add1/1  "motor torque"
  rotor resistor1/1 -> current/1, motor constant1/1  "current"

== system JenaFox_NCm_visualisation/motor model/hip_motor_right ==
  note: IC_phi_motor
  note: IC_v_motor
  note: due to neglectible inductivity the
      | PT1 - transfer function is reduced to an
      | proportional transfer function
      | (Modellbildung und Simulation dynamischer Systeme, S.122)
  U : Inport
  phi_motor : Inport  Port=2
  Add1 : Sum  Inputs=+--
  M_func_hip1 : Lookup  InputValues=[-10^10 -hip_na -0.001 0 0.001 hip_na 10^10]  Table=[-hip_Mrg -hip_Mrg -hip_Mrhg 0 hip_Mrhg hip_Mrg hip_Mrg]
  Radians to Degrees : simulink_extras/Transformations/Radians to Degrees
  Sum1 : Sum  Inputs=|+-
  elastic coupling : Sum  Inputs=+-
  elasticity : Gain  Gain=c_coupling_hip
  gearhead : Gain  Gain=hip_i
  gearhead1 : Gain  Gain=hip_i
  motor constant 1 : Gain  Gain=hip_k
  motor constant1 : Gain  Gain=hip_k
  motor interia : Gain  Gain=1/hip_Jm
  position : Integrator  InitialCondition=IC_motor_hip_r  ContinuousStateAttributes='position_hip'
  rotor resistor1 : Gain  Gain=1/hip_Ra
  speed : Integrator  InitialCondition=IC_v_motor_hip  ContinuousStateAttributes='speed_hip'
  motor_torque : Outport
  current : Outport  Port=2
  wires:
  elasticity/1 -> motor_torque/1, gearhead1/1  "coupling torque"
  gearhead1/1 -> Add1/3
  phi_motor/1 -> elastic coupling/2
  U/1 -> Sum1/1
  Radians to Degrees/1 -> gearhead/1  "position in °"
  gearhead/1 -> elastic coupling/1
  elastic coupling/1 -> elasticity/1
  position/1 -> Radians to Degrees/1  "position"
  motor constant 1/1 -> Sum1/2  "inductive voltage"
  speed/1 -> motor constant 1/1, M_func_hip1/1, position/1  "motor speed"
  Sum1/1 -> rotor resistor1/1
  motor interia/1 -> speed/1  "acceleration"
  Add1/1 -> motor interia/1
  M_func_hip1/1 -> Add1/2  "friction torque"
  motor constant1/1 -> Add1/1  "motor torque"
  rotor resistor1/1 -> current/1, motor constant1/1  "current"

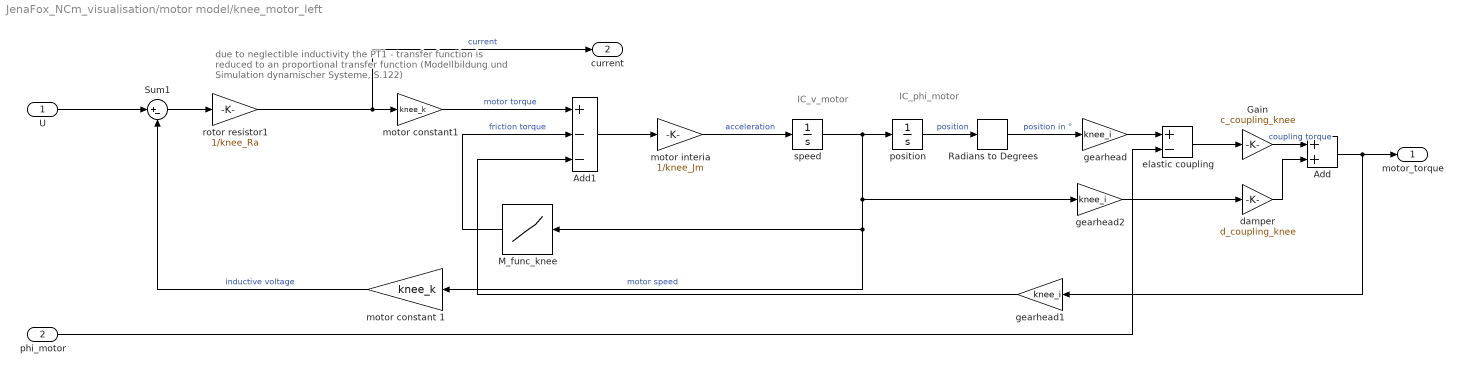
== system JenaFox_NCm_visualisation/motor model/knee_motor_left ==
  note: due to neglectible inductivity the
      | PT1 - transfer function is reduced to an
      | proportional transfer function
      | (Modellbildung und Simulation dynamischer Systeme, S.122)
  note: IC_v_motor
  note: IC_phi_motor
  U : Inport
  phi_motor : Inport  Port=2
  Add : Sum
  Add1 : Sum  Inputs=+--
  Gain : Gain  Gain=c_coupling_knee
  M_func_knee : Lookup  InputValues=[-10^10 -knee_na -0.001 0 0.001 knee_na 10^10]  Table=[-knee_Mrg -knee_Mrg -knee_Mrhg 0 knee_Mrhg knee_Mrg knee_Mrg]
  Radians to Degrees : simulink_extras/Transformations/Radians to Degrees
  Sum1 : Sum  Inputs=|+-
  damper : Gain  Gain=d_coupling_knee
  elastic coupling : Sum  Inputs=+-
  gearhead : Gain  Gain=knee_i
  gearhead1 : Gain  Gain=knee_i
  gearhead2 : Gain  Gain=knee_i
  motor constant 1 : Gain  Gain=knee_k
  motor constant1 : Gain  Gain=knee_k
  motor interia : Gain  Gain=1/knee_Jm
  position : Integrator  InitialCondition=IC_motor_knee_l  ContinuousStateAttributes='position_hip'
  rotor resistor1 : Gain  Gain=1/knee_Ra
  speed : Integrator  InitialCondition=IC_v_motor_knee  ContinuousStateAttributes='speed_hip'
  motor_torque : Outport
  current : Outport  Port=2
  wires:
  gearhead1/1 -> Add1/3
  rotor resistor1/1 -> motor constant1/1, current/1  "current"
  motor constant1/1 -> Add1/1  "motor torque"
  M_func_knee/1 -> Add1/2  "friction torque"
  Add1/1 -> motor interia/1
  motor interia/1 -> speed/1  "acceleration"
  Sum1/1 -> rotor resistor1/1
  speed/1 -> position/1, M_func_knee/1, motor constant 1/1, gearhead2/1  "motor speed"
  position/1 -> Radians to Degrees/1  "position"
  elastic coupling/1 -> Gain/1
  gearhead/1 -> elastic coupling/1
  Radians to Degrees/1 -> gearhead/1  "position in °"
  U/1 -> Sum1/1
  phi_motor/1 -> elastic coupling/2
  motor constant 1/1 -> Sum1/2  "inductive voltage"
  Gain/1 -> Add/1  "coupling torque"
  Add/1 -> motor_torque/1, gearhead1/1
  gearhead2/1 -> damper/1
  damper/1 -> Add/2

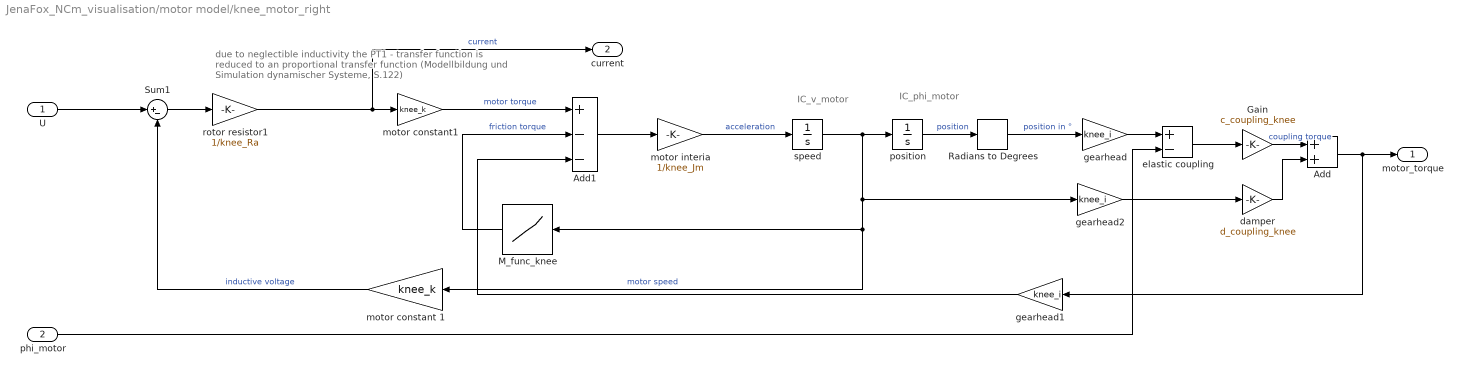
== system JenaFox_NCm_visualisation/motor model/knee_motor_right ==
  note: due to neglectible inductivity the
      | PT1 - transfer function is reduced to an
      | proportional transfer function
      | (Modellbildung und Simulation dynamischer Systeme, S.122)
  note: IC_v_motor
  note: IC_phi_motor
  U : Inport
  phi_motor : Inport  Port=2
  Add : Sum
  Add1 : Sum  Inputs=+--
  Gain : Gain  Gain=c_coupling_knee
  M_func_knee : Lookup  InputValues=[-10^10 -knee_na -0.001 0 0.001 knee_na 10^10]  Table=[-knee_Mrg -knee_Mrg -knee_Mrhg 0 knee_Mrhg knee_Mrg knee_Mrg]
  Radians to Degrees : simulink_extras/Transformations/Radians to Degrees
  Sum1 : Sum  Inputs=|+-
  damper : Gain  Gain=d_coupling_knee
  elastic coupling : Sum  Inputs=+-
  gearhead : Gain  Gain=knee_i
  gearhead1 : Gain  Gain=knee_i
  gearhead2 : Gain  Gain=knee_i
  motor constant 1 : Gain  Gain=knee_k
  motor constant1 : Gain  Gain=knee_k
  motor interia : Gain  Gain=1/knee_Jm
  position : Integrator  InitialCondition=IC_phi_motor_knee  ContinuousStateAttributes='position_hip'
  rotor resistor1 : Gain  Gain=1/knee_Ra
  speed : Integrator  InitialCondition=IC_v_motor_knee  ContinuousStateAttributes='speed_hip'
  motor_torque : Outport
  current : Outport  Port=2
  wires:
  gearhead1/1 -> Add1/3
  rotor resistor1/1 -> motor constant1/1, current/1  "current"
  motor constant1/1 -> Add1/1  "motor torque"
  M_func_knee/1 -> Add1/2  "friction torque"
  Add1/1 -> motor interia/1
  motor interia/1 -> speed/1  "acceleration"
  Sum1/1 -> rotor resistor1/1
  speed/1 -> position/1, M_func_knee/1, motor constant 1/1, gearhead2/1  "motor speed"
  position/1 -> Radians to Degrees/1  "position"
  elastic coupling/1 -> Gain/1
  gearhead/1 -> elastic coupling/1
  Radians to Degrees/1 -> gearhead/1  "position in °"
  U/1 -> Sum1/1
  phi_motor/1 -> elastic coupling/2
  motor constant 1/1 -> Sum1/2  "inductive voltage"
  Gain/1 -> Add/1  "coupling torque"
  Add/1 -> motor_torque/1, gearhead1/1
  gearhead2/1 -> damper/1
  damper/1 -> Add/2

== system JenaFox_NCm_visualisation/Subsystem/Ground Contact Model/Ground Friction Model ==
  note: Horizontal Ground Friction Model
  note: Vertical Ground Stiction Model
  dy [m] : Inport
  vy [m/s] : Inport  Port=2
  x [m] : Inport  Port=3
  vx [m/s] : Inport  Port=4
  Contact! : EnablePort  StatesWhenEnabling=reset  PropagateVarSize=During execution
  Data Type Conversion : DataTypeConversion  OutDataTypeStr=double
  Friction Switch : Subsystem
  Gain3 : Gain  Gain=k_gy
  Gain4 : Gain  Gain=1/v_gy_max
  Logical Operator : Logic  Operator=NOT  AllPortsSameDT=off  OutDataTypeStr=boolean
  Mux1 : Mux  Inputs=2
  Sum1 : Sum
  X-Axis Kinetic Friction Model : Subsystem
  X-Axis Static Friction Model : Subsystem
  Y-Axis Ground Force : Fcn  Expr="- u(1)  *  (1-u(2)) * (u(2)<1)"
  Fy_Ground[N] : Outport  OutputWhenDisabled=reset  InitialOutput=0
      settings: AttributesFormatString=initial = '%<InitialOutput>'\nwhen disabled = '%<OutputWhenDisabled>'
  Fx_Friction [N] : Outport  Port=2  OutputWhenDisabled=reset  InitialOutput=0
      settings: AttributesFormatString=initial = '%<InitialOutput>'\nwhen\ndisabled\n'%<OutputWhenDisabled>'
  Stiction! : Outport  Port=3  OutputWhenDisabled=reset  InitialOutput=0
      settings: AttributesFormatString=initial = '%<InitialOutput>'\nwhen\ndisabled\n'%<OutputWhenDisabled>'
  wires:
  dy [m]/1 -> Gain3/1
  vy [m/s]/1 -> Gain4/1
  x [m]/1 -> X-Axis Static Friction Model/2(pos [m]), X-Axis Kinetic Friction Model/1(pos [m])
  vx [m/s]/1 -> X-Axis Static Friction Model/3(vel [m/s]), X-Axis Kinetic Friction Model/2(vel [m/s])
  X-Axis Kinetic Friction Model/1(posFP [m]) -> X-Axis Static Friction Model/4(posFP [m])
  X-Axis Kinetic Friction Model/3(F_Slide [N]) -> Sum1/2
  X-Axis Static Friction Model/1(F_Stick [N]) -> Sum1/1
  Sum1/1 -> Fx_Friction [N]/1
  Friction Switch/1(Stiction) -> X-Axis Static Friction Model/Enable, Logical Operator/1, Data Type Conversion/1
  X-Axis Static Friction Model/2(Sliding!) -> Friction Switch/1(Slide!)
  X-Axis Kinetic Friction Model/2(Stiction!) -> Friction Switch/2(Stick!)
  Logical Operator/1 -> X-Axis Kinetic Friction Model/Enable
  Data Type Conversion/1 -> Stiction!/1
  Mux1/1 -> Y-Axis Ground Force/1
  Gain3/1 -> Mux1/1
  Gain4/1 -> Mux1/2
  Y-Axis Ground Force/1 -> Fy_Ground[N]/1, X-Axis Static Friction Model/1(F_Normal [N]), X-Axis Kinetic Friction Model/3(F_Normal [N])

== system JenaFox_NCm_visualisation/Subsystem/Ground Contact Model1/Ground Friction Model ==
  note: Horizontal Ground Friction Model
  note: Vertical Ground Stiction Model
  dy [m] : Inport
  vy [m/s] : Inport  Port=2
  x [m] : Inport  Port=3
  vx [m/s] : Inport  Port=4
  Contact! : EnablePort  StatesWhenEnabling=reset  PropagateVarSize=During execution
  Data Type Conversion : DataTypeConversion  OutDataTypeStr=double
  Friction Switch : Subsystem
  Gain3 : Gain  Gain=k_gy
  Gain4 : Gain  Gain=1/v_gy_max
  Logical Operator : Logic  Operator=NOT  AllPortsSameDT=off  OutDataTypeStr=boolean
  Mux1 : Mux  Inputs=2
  Sum1 : Sum
  X-Axis Kinetic Friction Model : Subsystem
  X-Axis Static Friction Model : Subsystem
  Y-Axis Ground Force : Fcn  Expr="- u(1)  *  (1-u(2)) * (u(2)<1)"
  Fy_Ground[N] : Outport  OutputWhenDisabled=reset  InitialOutput=0
      settings: AttributesFormatString=initial = '%<InitialOutput>'\nwhen disabled = '%<OutputWhenDisabled>'
  Fx_Friction [N] : Outport  Port=2  OutputWhenDisabled=reset  InitialOutput=0
      settings: AttributesFormatString=initial = '%<InitialOutput>'\nwhen\ndisabled\n'%<OutputWhenDisabled>'
  Stiction! : Outport  Port=3  OutputWhenDisabled=reset  InitialOutput=0
      settings: AttributesFormatString=initial = '%<InitialOutput>'\nwhen\ndisabled\n'%<OutputWhenDisabled>'
  wires:
  dy [m]/1 -> Gain3/1
  vy [m/s]/1 -> Gain4/1
  x [m]/1 -> X-Axis Static Friction Model/2(pos [m]), X-Axis Kinetic Friction Model/1(pos [m])
  vx [m/s]/1 -> X-Axis Static Friction Model/3(vel [m/s]), X-Axis Kinetic Friction Model/2(vel [m/s])
  X-Axis Kinetic Friction Model/1(posFP [m]) -> X-Axis Static Friction Model/4(posFP [m])
  X-Axis Kinetic Friction Model/3(F_Slide [N]) -> Sum1/2
  X-Axis Static Friction Model/1(F_Stick [N]) -> Sum1/1
  Sum1/1 -> Fx_Friction [N]/1
  Friction Switch/1(Stiction) -> X-Axis Static Friction Model/Enable, Logical Operator/1, Data Type Conversion/1
  X-Axis Static Friction Model/2(Sliding!) -> Friction Switch/1(Slide!)
  X-Axis Kinetic Friction Model/2(Stiction!) -> Friction Switch/2(Stick!)
  Logical Operator/1 -> X-Axis Kinetic Friction Model/Enable
  Data Type Conversion/1 -> Stiction!/1
  Mux1/1 -> Y-Axis Ground Force/1
  Gain3/1 -> Mux1/1
  Gain4/1 -> Mux1/2
  Y-Axis Ground Force/1 -> Fy_Ground[N]/1, X-Axis Static Friction Model/1(F_Normal [N]), X-Axis Kinetic Friction Model/3(F_Normal [N])

== system JenaFox_NCm_visualisation/Subsystem/knee_l/hard stop extension ==
  note: generate a positive torque to counteract flexion
      | beyond -90°
      | and negative torque to inhibit hyperextension beyond 0°
  phi : Inport
  vphi : Inport  Port=2
  Enable : EnablePort  PropagateVarSize=During execution
  Fcn : Fcn  Expr=c_hs*(0-u[1])-d_hs*u[2]
  Mux : Mux  Inputs=2
  T_hs : Outport  OutputWhenDisabled=reset  InitialOutput=0
  wires:
  phi/1 -> Mux/1
  vphi/1 -> Mux/2
  Mux/1 -> Fcn/1
  Fcn/1 -> T_hs/1

== system JenaFox_NCm_visualisation/Subsystem/knee_l/hard stop flexion ==
  note: generate a positive torque to counteract flexion
      | beyond -90°
      | and negative torque to inhibit hyperextension beyond 0°
  phi : Inport
  vphi : Inport  Port=2
  Enable : EnablePort  PropagateVarSize=During execution
  Fcn : Fcn  Expr=c_hs*(-92-u[1])-d_hs*u[2]
  Mux : Mux  Inputs=2
  T_hs : Outport  OutputWhenDisabled=reset  InitialOutput=0
  wires:
  Fcn/1 -> T_hs/1
  Mux/1 -> Fcn/1
  vphi/1 -> Mux/2
  phi/1 -> Mux/1

== system JenaFox_NCm_visualisation/Subsystem/knee_r/hard stop extension ==
  note: generate a positive torque to counteract flexion
      | beyond -90°
      | and negative torque to inhibit hyperextension beyond 0°
  phi : Inport
  vphi : Inport  Port=2
  Enable : EnablePort  PropagateVarSize=During execution
  Fcn : Fcn  Expr=c_hs*(0-u[1])-d_hs*u[2]
  Mux : Mux  Inputs=2
  T_hs : Outport  OutputWhenDisabled=reset  InitialOutput=0
  wires:
  phi/1 -> Mux/1
  vphi/1 -> Mux/2
  Mux/1 -> Fcn/1
  Fcn/1 -> T_hs/1

== system JenaFox_NCm_visualisation/Subsystem/knee_r/hard stop flexion ==
  note: generate a positive torque to counteract flexion
      | beyond -90°
      | and negative torque to inhibit hyperextension beyond 0°
  phi : Inport
  vphi : Inport  Port=2
  Enable : EnablePort  PropagateVarSize=During execution
  Fcn : Fcn  Expr=c_hs*(-92-u[1])-d_hs*u[2]
  Mux : Mux  Inputs=2
  T_hs : Outport  OutputWhenDisabled=reset  InitialOutput=0
  wires:
  Fcn/1 -> T_hs/1
  Mux/1 -> Fcn/1
  vphi/1 -> Mux/2
  phi/1 -> Mux/1

== system JenaFox_NCm_visualisation/Subsystem/simulation terminator/Subsystem ==
  error : Inport
  x : Inport  Port=2
  Compare To Constant5 : simulink/Logic and Bit Operations/Compare To Constant  relop=>=  const=5  OutDataTypeStr=boolean
  Constant : Constant  Value=errorswitch
  Constant1 : Constant  Value=stop5m
  Logical Operator : Logic  Operator=OR  AllPortsSameDT=off  OutDataTypeStr=boolean
  Logical Operator1 : Logic  AllPortsSameDT=off  OutDataTypeStr=boolean
  Logical Operator2 : Logic  AllPortsSameDT=off  OutDataTypeStr=boolean
  Stop Simulation1 : Stop
  wires:
  x/1 -> Compare To Constant5/1
  Logical Operator2/1 -> Logical Operator/2
  Constant/1 -> Logical Operator1/1
  error/1 -> Logical Operator1/2
  Logical Operator1/1 -> Logical Operator/1
  Logical Operator/1 -> Stop Simulation1/1
  Constant1/1 -> Logical Operator2/1
  Compare To Constant5/1 -> Logical Operator2/2

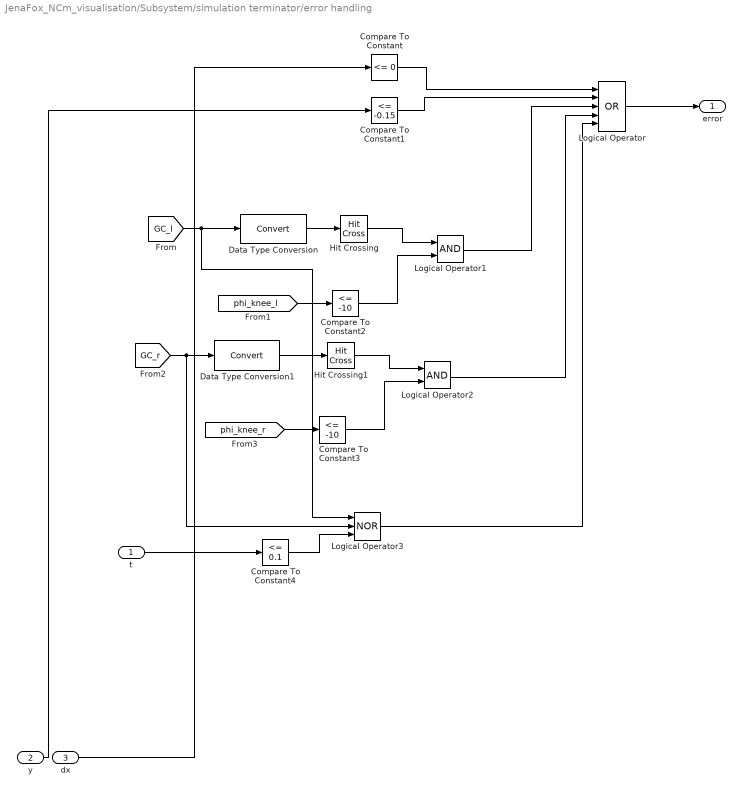
== system JenaFox_NCm_visualisation/Subsystem/simulation terminator/error handling ==
  t : Inport
  y : Inport  Port=2
  dx : Inport  Port=3
  Compare To Constant : simulink/Logic and Bit Operations/Compare To Constant  relop=<=  const=0  OutDataTypeStr=boolean
  Compare To Constant1 : simulink/Logic and Bit Operations/Compare To Constant  relop=<=  const=-0.15  OutDataTypeStr=boolean
  Compare To Constant2 : simulink/Logic and Bit Operations/Compare To Constant  relop=<=  const=-10  OutDataTypeStr=boolean
  Compare To Constant3 : simulink/Logic and Bit Operations/Compare To Constant  relop=<=  const=-10  OutDataTypeStr=boolean
  Compare To Constant4 : simulink/Logic and Bit Operations/Compare To Constant  relop=<=  const=0.1  OutDataTypeStr=boolean
  Data Type Conversion : DataTypeConversion
  Data Type Conversion1 : DataTypeConversion
  Hit Crossing : HitCross  HitCrossingOffset=0.5  HitCrossingDirection=rising
  Hit Crossing1 : HitCross  HitCrossingOffset=0.5  HitCrossingDirection=rising
  Logical Operator : Logic  Operator=OR  Inputs=5  AllPortsSameDT=off  OutDataTypeStr=boolean
  Logical Operator1 : Logic  AllPortsSameDT=off  OutDataTypeStr=boolean
  Logical Operator2 : Logic  AllPortsSameDT=off  OutDataTypeStr=boolean
  Logical Operator3 : Logic  Operator=NOR  Inputs=3  AllPortsSameDT=off  OutDataTypeStr=boolean
  error : Outport
  wires:
  [phi_knee_r] -> Compare To Constant3/1
  [GC_r] -> Logical Operator3/2, Data Type Conversion1/1
  Compare To Constant3/1 -> Logical Operator2/2
  Logical Operator1/1 -> Logical Operator/3
  Hit Crossing/1 -> Logical Operator1/1
  Logical Operator3/1 -> Logical Operator/5
  Compare To Constant2/1 -> Logical Operator1/2
  [phi_knee_l] -> Compare To Constant2/1
  Hit Crossing1/1 -> Logical Operator2/1
  Data Type Conversion1/1 -> Hit Crossing1/1
  y/1 -> Compare To Constant1/1
  t/1 -> Compare To Constant4/1
  Logical Operator2/1 -> Logical Operator/4
  Data Type Conversion/1 -> Hit Crossing/1
  Compare To Constant4/1 -> Logical Operator3/3
  [GC_l] -> Logical Operator3/1, Data Type Conversion/1
  Logical Operator/1 -> error/1
  Compare To Constant1/1 -> Logical Operator/2
  dx/1 -> Compare To Constant/1
  Compare To Constant/1 -> Logical Operator/1

== system JenaFox_NCm_visualisation/Subsystem/simulation terminator/time of termination ==
  error : Inport
  t : Inport  Port=2
  x : Inport  Port=3
  Divide : Product  Inputs=*/
  Gain : Gain  Gain=5
  Mux1 : Mux  Inputs=2
  Switch : Switch  Criteria=u2 > Threshold  Threshold=0.5
  To Workspace : ToWorkspace  VariableName=t_end  SampleTime=-1
      settings: MaxDataPoints=1
  wires:
  x/1 -> Divide/2, Mux1/2
  error/1 -> Switch/2
  t/1 -> Switch/3, Gain/1
  Mux1/1 -> To Workspace/1
  Gain/1 -> Divide/1
  Switch/1 -> Mux1/1
  Divide/1 -> Switch/1

== system JenaFox_NCm_visualisation/Subsystem/Ground Contact Model/Ground Friction Model/Friction Switch ==
  note: Static/Kinetic Friction Switch
  Slide! : Inport
  Stick! : Inport  Port=2
  Memory : Memory
  S-R Flip-Flop : simulink_extras/Flip Flops/S-R Flip-Flop  initial_condition=1
  Terminator : Terminator
  Stiction : Outport
  wires:
  S-R Flip-Flop/1 -> Memory/1
  S-R Flip-Flop/2 -> Terminator/1
  Stick!/1 -> S-R Flip-Flop/1
  Slide!/1 -> S-R Flip-Flop/2
  Memory/1 -> Stiction/1
